simulink model "sampleModel1420_5"  (R2023a)
settings: Solver=VariableStepAuto  StartTime=0.0  StopTime=10.0  RelTol=1e-3
libraries: hdlsllib x5, simulink x2
settings Model: Creator=user1  LastModifiedBy=user1

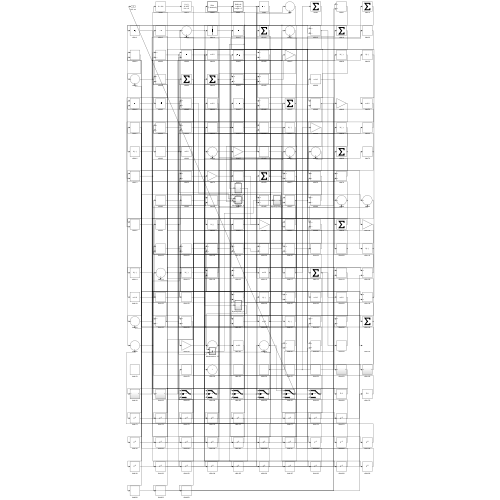
[thumbnail: Simulink's stored preview of the top-level diagram]
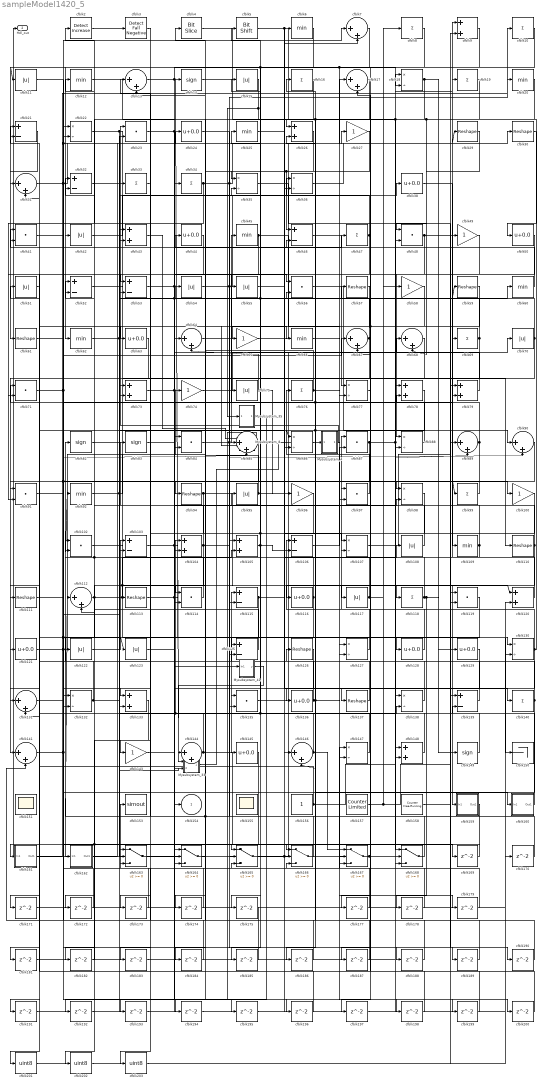
== system sampleModel1420_5 ==
  Mysubsystem_33 : Subsystem  TreatAsAtomicUnit=on  RTWFcnName=Mysubsystem_33
      settings: RTWFcnNameOpts=User specified  RTWFileNameOpts=Use function name
  Mysubsystem_35 : Subsystem  TreatAsAtomicUnit=on  RTWFcnName=Mysubsystem_35
      settings: RTWFcnNameOpts=User specified  RTWFileNameOpts=Use function name
  Mysubsystem_4 : Subsystem  TreatAsAtomicUnit=on  RTWFcnName=Mysubsystem_4
      settings: RTWFcnNameOpts=User specified  RTWFileNameOpts=Use function name
  Mysubsystem_41 : Subsystem  TreatAsAtomicUnit=on  RTWFcnName=Mysubsystem_41
      settings: RTWFcnNameOpts=User specified  RTWFileNameOpts=Use function name
  Mysubsystem_8 : Subsystem  TreatAsAtomicUnit=on  RTWFcnName=Mysubsystem_8
      settings: RTWFcnNameOpts=User specified  RTWFileNameOpts=Use function name
  cfblk{8,10,16,19,33..34,47,69,76,99,118,140} (12 alike) : Sum  Inputs=+  OutDataTypeStr=uint8
  cfblk{27,49,58,65,74,96,100,143} (8 alike) : Gain  OutDataTypeStr=uint8
  cfblk{23,41,48,56,71,84,87,91,97,102,114,119,135} (13 alike) : DotProduct  OutDataTypeStr=uint8
  cfblk{21,32,46,52..53,103,106,115,125,139} (10 alike) : Sum  Inputs=+-  OutDataTypeStr=uint8
  cfblk{9,26,43,73,78..79,104..105,120,133,148} (11 alike) : Sum  OutDataTypeStr=uint8
  cfblk{18,22,35..36,77,86,88,98,107,127,130,132,138,147} (14 alike) : Product  Inputs=*/  OutDataTypeStr=uint8  RndMeth=Zero  SaturateOnIntegerOverflow=on
  cfblk{11,15,42,51,54..55,70,75,95,108,117,122..123} (13 alike) : Abs  OutDataTypeStr=uint8  SaturateOnIntegerOverflow=off
  cfblk{6,12,20,25,45,60,62,66,92,109} (10 alike) : MinMax  OutDataTypeStr=uint8
  cfblk{29..30,57,59,61,94,110..111,113,126,137} (11 alike) : Reshape
  cfblk{7,13,17,31,64,67..68,85,89..90,112,131,141,144,146} (15 alike) : Sum  Inputs=|++  OutDataTypeStr=uint8
  cfblk{24,38,44,50,63,116,121,128..129,136,145} (11 alike) : Bias  Bias=0.0  SaturateOnIntegerOverflow=off
  cfblk{14,82..83,149} (4 alike) : Signum
  cfblk150 : Terminator
  cfblk151 : Scope
      settings: Floating=on
  cfblk153 : ToWorkspace  VariableName=simout  SaveFormat=Timeseries  SampleTime=-1
  cfblk155 : Scope
      settings: Floating=on
  cfblk156 : Constant  OutDataTypeStr=uint8  SampleTime=-1
  cfblk157 : hdlsllib/Sources/Counter Limited  uplimit=7  tsamp=-1
  cfblk158 : hdlsllib/Sources/Counter Free-Running  NumBits=16  tsamp=-1
  cfblk159 : Subsystem
      settings: LibrarySourceBlock=|
      | hdlsllib/Ports &
      | Subsystems/Subsystem
  cfblk160 : Subsystem
      settings: LibrarySourceBlock=|
      | hdlsllib/Ports &
      | Subsystems/Subsystem
  cfblk161 : Subsystem
      settings: LibrarySourceBlock=|
      | hdlsllib/Ports &
      | Subsystems/Subsystem
  cfblk162 : Subsystem
      settings: LibrarySourceBlock=|
      | hdlsllib/Ports &
      | Subsystems/Subsystem
  cfblk{163..168} (6 alike) : Switch  OutDataTypeStr=uint8  SaturateOnIntegerOverflow=off  InputSameDT=off
  cfblk{169..175,177..179,181..200} (30 alike) : Delay  SampleTime=1
  cfblk2 : simulink/Logic and Bit Operations/Detect Increase  vinit=0.0  OutDataTypeStr=uint8
      settings: LibrarySourceBlock=|
      | hdlsllib/Logic and Bit
      | Operations/Detect
      | Increase
  cfblk201 : DataTypeConversion  OutDataTypeStr=uint8  SaturateOnIntegerOverflow=off  RndMeth=Floor
  cfblk202 : DataTypeConversion  OutDataTypeStr=uint8  SaturateOnIntegerOverflow=off  RndMeth=Floor
  cfblk203 : DataTypeConversion  OutDataTypeStr=uint8  SaturateOnIntegerOverflow=off  RndMeth=Floor
  cfblk3 : hdlsllib/Logic and Bit Operations/Detect Fall Negative  vinit=0  OutDataTypeStr=uint8
  cfblk4 : hdlsllib/Logic and Bit Operations/Bit Slice  lidx=7  ridx=0
  cfblk5 : hdlsllib/Logic and Bit Operations/Bit Shift  mode=Shift Left Logical  N=0
  cfblk154 : Outport  OutDataTypeStr=uint8  VectorParamsAs1DForOutWhenUnconnected=off
  Hdl_out : Outport  Port=2  OutDataTypeStr=uint8
  wires:
  cfblk165/1 -> cfblk70/1, cfblk108/1
  cfblk140/1 -> cfblk153/1, cfblk126/1
  cfblk144/1 -> cfblk166/1, cfblk41/2
  cfblk139/1 -> cfblk115/1
  cfblk6/1 -> cfblk61/1
  cfblk75/1 -> cfblk96/1, cfblk64/2
  cfblk162/1(Out1) -> cfblk27/1
  cfblk59/1 -> Mysubsystem_8/2(In2), cfblk197/1
  cfblk54/1 -> cfblk38/1, cfblk188/1
  cfblk138/1 -> cfblk82/1
  cfblk161/1(Out1) -> cfblk10/1
  cfblk62/1 -> cfblk130/1, cfblk60/1
  cfblk94/1 -> cfblk159/1(In1), cfblk183/1
  cfblk10/1 -> cfblk62/1
  cfblk127/1 -> cfblk87/1
  cfblk130/1 -> cfblk26/1, cfblk164/3, cfblk67/2
  cfblk115/1 -> cfblk162/1(In1), cfblk7/2
  cfblk22/1 -> cfblk118/1, cfblk86/2
  cfblk70/1 -> cfblk141/1, cfblk53/2
  cfblk48/1 -> cfblk88/1, cfblk190/1
  cfblk23/1 -> cfblk144/1, cfblk167/3
  cfblk116/1 -> cfblk43/1, cfblk191/1
  cfblk63/1 -> cfblk161/1(In1)
  cfblk97/1 -> cfblk76/1
  cfblk146/1 -> cfblk25/1, cfblk21/1, cfblk167/1
  cfblk56/1 -> cfblk90/1
  cfblk148/1 -> cfblk104/1, cfblk43/2
  cfblk121/1 -> cfblk74/1, cfblk67/1
  cfblk16/1 -> cfblk53/1
  cfblk110/1 -> cfblk83/1, cfblk136/1
  cfblk95/1 -> cfblk44/1, cfblk98/1
  cfblk4/1 -> cfblk127/1
  cfblk168/1 -> cfblk112/1, cfblk114/2
  cfblk87/1 -> cfblk89/2, cfblk19/1, cfblk175/1
  cfblk5/1 -> cfblk168/1, cfblk107/1
  cfblk117/1 -> cfblk92/1, cfblk2/1, cfblk58/1
  cfblk26/1 -> cfblk165/1
  cfblk109/1 -> cfblk97/1, cfblk107/2
  cfblk85/1 -> cfblk121/1
  cfblk46/1 -> cfblk77/1
  cfblk120/1 -> cfblk9/1
  cfblk104/1 -> cfblk73/2, cfblk122/1, cfblk20/1
  cfblk50/1 -> cfblk85/1
  cfblk88/1 -> cfblk45/1
  cfblk57/1 -> cfblk91/1
  cfblk12/1 -> cfblk64/1
  cfblk51/1 -> cfblk131/1
  cfblk125/1 -> cfblk71/1
  cfblk106/1 -> cfblk87/2
  cfblk65/1 -> cfblk17/1
  cfblk2/1 -> cfblk3/1
  cfblk67/1 -> cfblk115/2, cfblk15/1
  cfblk112/1 -> cfblk147/2, cfblk34/1, cfblk12/1
  cfblk122/1 -> cfblk103/1
  cfblk34/1 -> cfblk55/1, cfblk18/1, cfblk71/2
  cfblk11/1 -> cfblk164/2
  cfblk38/1 -> cfblk109/1
  cfblk149/1 -> cfblk54/1
  cfblk64/1 -> cfblk66/1
  cfblk17/1 -> cfblk146/2, cfblk173/1
  cfblk47/1 -> cfblk91/2, cfblk13/1
  cfblk123/1 -> cfblk154/1
  cfblk163/1 -> cfblk105/2
  cfblk156/1 -> cfblk131/2, cfblk48/2
  cfblk90/1 -> cfblk132/2
  cfblk31/1 -> cfblk14/1, cfblk7/1
  cfblk158/1 -> cfblk139/1
  cfblk45/1 -> cfblk97/2, cfblk103/2
  cfblk159/1(Out1) -> cfblk181/1, cfblk182/1
  cfblk27/1 -> cfblk46/1, cfblk184/1
  cfblk108/1 -> cfblk52/1
  cfblk83/1 -> cfblk36/1, cfblk59/1
  cfblk103/1 -> cfblk150/1, cfblk57/1
  cfblk86/1 -> cfblk100/1
  cfblk113/1 -> cfblk128/1, cfblk98/2
  cfblk84/1 -> cfblk90/2, cfblk79/2
  cfblk166/1 -> cfblk33/1
  cfblk15/1 -> Mysubsystem_35/1(In1), cfblk193/1
  cfblk135/1 -> cfblk137/1
  cfblk36/1 -> cfblk30/1
  cfblk92/1 -> cfblk24/1, cfblk167/2
  cfblk132/1 -> cfblk51/1, cfblk138/2
  cfblk29/1 -> cfblk48/1
  cfblk76/1 -> cfblk13/2, cfblk179/1
  cfblk79/1 -> cfblk65/1
  cfblk105/1 -> cfblk5/1, cfblk106/2
  cfblk61/1 -> cfblk123/1, cfblk160/1(In1), cfblk99/1
  cfblk102/1 -> cfblk145/1, cfblk120/1
  cfblk98/1 -> cfblk135/1, cfblk125/2
  cfblk69/1 -> cfblk4/1, cfblk35/2, cfblk194/1
  cfblk21/1 -> cfblk31/1
  cfblk73/1 -> cfblk69/1, cfblk195/1
  cfblk58/1 -> cfblk78/1
  cfblk167/1 -> cfblk138/1, Hdl_out/1
  cfblk141/1 -> cfblk163/2, cfblk113/1
  cfblk74/1 -> cfblk68/1
  cfblk52/1 -> cfblk110/1
  cfblk71/1 -> cfblk22/2, cfblk29/1, cfblk85/2
  cfblk82/1 -> cfblk75/1
  cfblk164/1 -> cfblk84/2
  cfblk33/1 -> cfblk63/1
  cfblk107/1 -> cfblk49/1
  cfblk30/1 -> cfblk50/1
  cfblk53/1 -> cfblk56/1, cfblk199/1
  cfblk131/1 -> cfblk78/2
  cfblk99/1 -> cfblk94/1
  cfblk96/1 -> cfblk133/1
  cfblk128/1 -> cfblk106/1
  cfblk13/1 -> Mysubsystem_41/1(In1), cfblk18/2
  cfblk114/1 -> cfblk52/2
  cfblk25/1 -> cfblk140/1
  cfblk19/1 -> cfblk125/1, cfblk68/2
  cfblk143/1 -> cfblk47/1
  cfblk89/1 -> cfblk32/1, cfblk56/2, cfblk135/2
  cfblk20/1 -> cfblk88/2, cfblk114/1
  cfblk9/1 -> cfblk11/1, cfblk35/1, cfblk127/2
  cfblk147/1 -> cfblk102/1
  cfblk24/1 -> cfblk77/2
  cfblk18/1 -> cfblk42/1, cfblk129/1
  cfblk68/1 -> cfblk86/1, cfblk116/1
  cfblk44/1 -> cfblk111/1
  cfblk35/1 -> cfblk89/1
  cfblk42/1 -> cfblk6/1
  cfblk100/1 -> cfblk143/1
  cfblk41/1 -> cfblk133/2
  cfblk136/1 -> cfblk16/1, cfblk200/1, cfblk95/1
  cfblk160/1(Out1) -> cfblk139/2
  cfblk60/1 -> cfblk41/1
  cfblk14/1 -> cfblk148/1
  cfblk55/1 -> cfblk36/2
  cfblk118/1 -> cfblk149/1, cfblk178/1, cfblk32/2
  cfblk157/1 -> cfblk9/2, cfblk8/1
  cfblk8/1 -> cfblk117/1
  cfblk137/1 -> cfblk46/2
  cfblk66/1 -> cfblk169/1
  cfblk169/1 -> cfblk165/2
  cfblk170/1 -> cfblk105/1
  cfblk78/1 -> cfblk171/1
  cfblk171/1 -> cfblk130/2
  cfblk133/1 -> cfblk172/1
  cfblk172/1 -> cfblk132/1
  cfblk173/1 -> cfblk163/1
  cfblk126/1 -> cfblk174/1
  cfblk174/1 -> cfblk112/2
  cfblk175/1 -> cfblk141/2
  cfblk77/1 -> cfblk177/1
  cfblk177/1 -> cfblk166/3
  cfblk178/1 -> cfblk147/1
  cfblk179/1 -> cfblk165/3
  cfblk181/1 -> cfblk144/2
  cfblk182/1 -> cfblk102/2
  cfblk183/1 -> cfblk148/2
  cfblk184/1 -> cfblk163/3
  cfblk7/1 -> cfblk185/1
  cfblk185/1 -> cfblk22/1
  cfblk129/1 -> cfblk186/1
  cfblk186/1 -> cfblk84/1
  cfblk49/1 -> cfblk187/1
  cfblk187/1 -> cfblk26/2
  cfblk188/1 -> cfblk104/2
  cfblk91/1 -> cfblk189/1
  cfblk189/1 -> cfblk73/1
  cfblk190/1 -> cfblk21/2
  cfblk191/1 -> cfblk164/1
  cfblk192/1 -> cfblk23/2
  cfblk193/1 -> cfblk120/2
  cfblk194/1 -> cfblk79/1
  cfblk195/1 -> cfblk146/1
  cfblk196/1 -> cfblk166/2
  cfblk197/1 -> cfblk168/3
  cfblk111/1 -> cfblk198/1
  cfblk198/1 -> cfblk168/2
  cfblk199/1 -> cfblk17/2
  cfblk200/1 -> cfblk31/2
  cfblk119/1 -> cfblk201/1
  cfblk201/1 -> cfblk170/1
  cfblk145/1 -> cfblk202/1
  cfblk202/1 -> cfblk119/1
  cfblk3/1 -> cfblk203/1
  cfblk203/1 -> cfblk119/2
  Mysubsystem_4/1(Out1) -> cfblk23/1
  cfblk43/1 -> Mysubsystem_8/1(In1)
  Mysubsystem_8/1(Out1) -> cfblk196/1
  cfblk32/1 -> Mysubsystem_33/2(In2)
  Mysubsystem_33/1(Out1) -> Mysubsystem_4/1(In1)
  Mysubsystem_35/1(Out1) -> cfblk192/1
  Mysubsystem_41/1(y) -> Mysubsystem_33/1(In1)

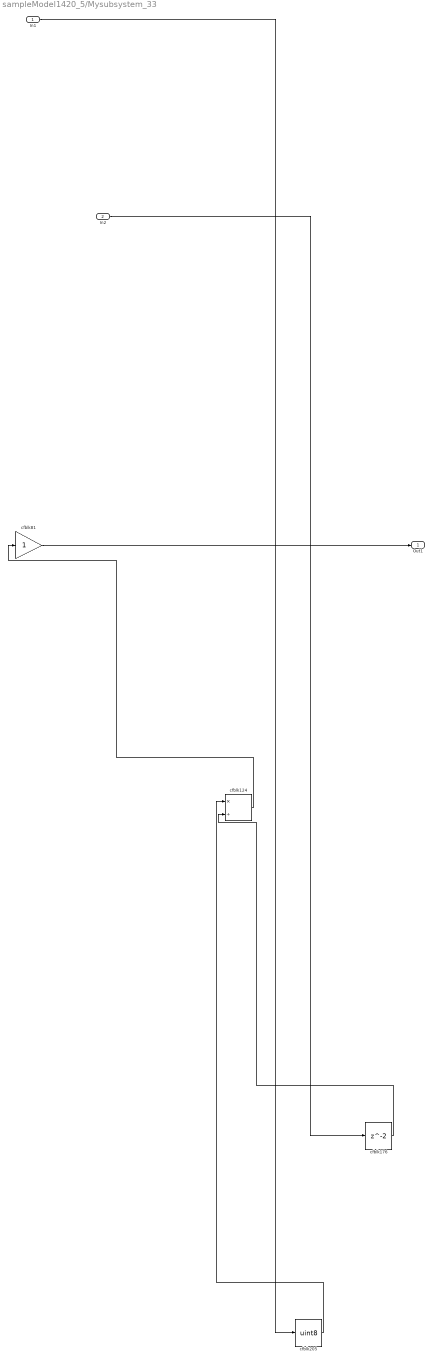
== system sampleModel1420_5/Mysubsystem_33 ==
  In1 : Inport
  In2 : Inport  Port=2
  cfblk124 : Product  Inputs=*/  RndMeth=Zero  SaturateOnIntegerOverflow=on
  cfblk176 : Delay  SampleTime=1
  cfblk205 : DataTypeConversion  OutDataTypeStr=uint8  SaturateOnIntegerOverflow=off  RndMeth=Floor
  cfblk81 : Gain
  Out1 : Outport
  wires:
  cfblk81/1 -> Out1/1
  cfblk205/1 -> cfblk124/1
  In2/1 -> cfblk176/1
  cfblk176/1 -> cfblk124/2
  cfblk124/1 -> cfblk81/1
  In1/1 -> cfblk205/1

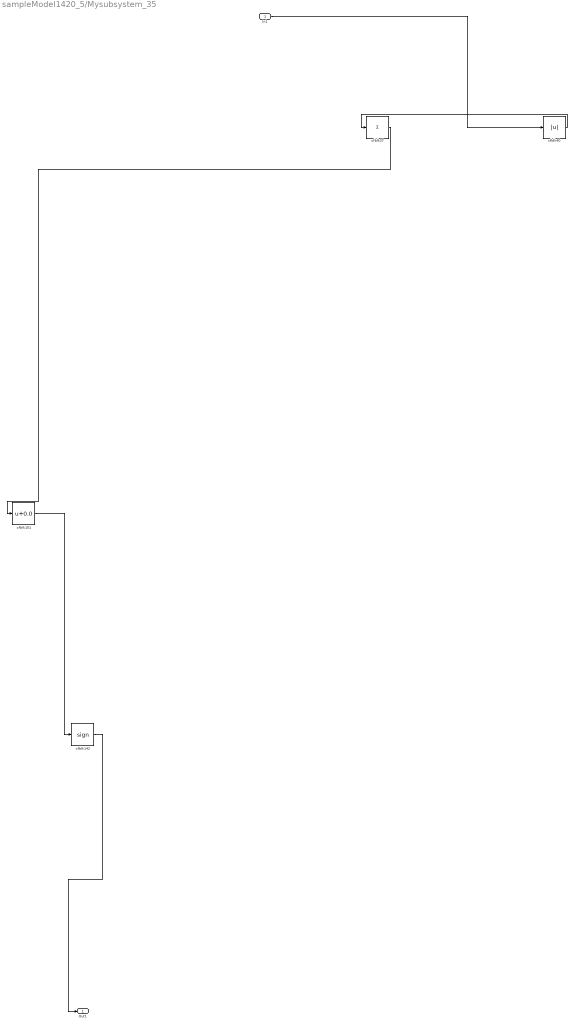
== system sampleModel1420_5/Mysubsystem_35 ==
  In1 : Inport
  cfblk101 : Bias  Bias=0.0  SaturateOnIntegerOverflow=off
  cfblk142 : Signum
  cfblk37 : Sum  Inputs=+
  cfblk40 : Abs  SaturateOnIntegerOverflow=off
  Out1 : Outport
  wires:
  cfblk37/1 -> cfblk101/1
  In1/1 -> cfblk40/1
  cfblk40/1 -> cfblk37/1
  cfblk101/1 -> cfblk142/1
  cfblk142/1 -> Out1/1

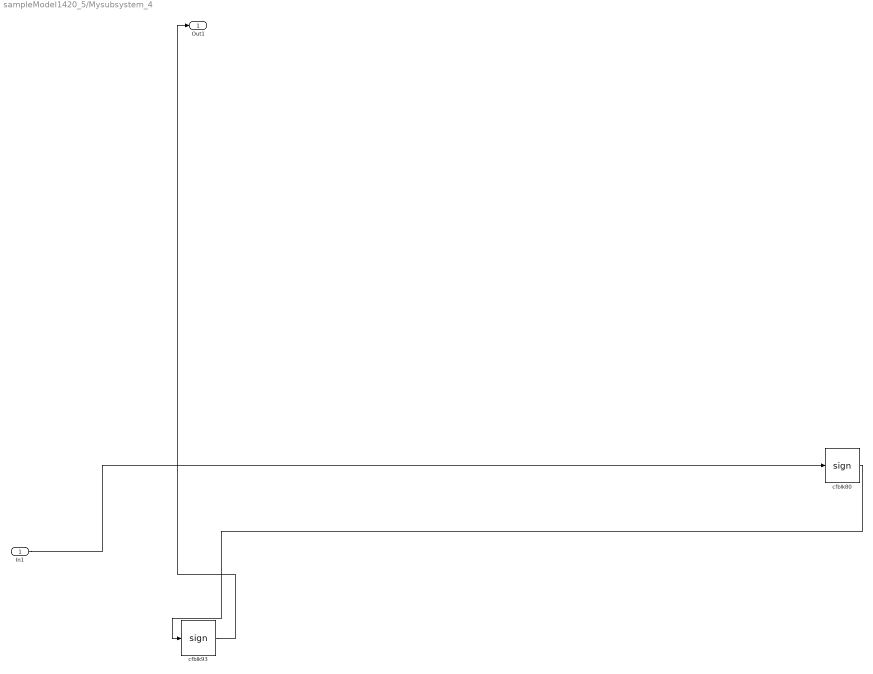
== system sampleModel1420_5/Mysubsystem_4 ==
  In1 : Inport
  cfblk80 : Signum
  cfblk93 : Signum
  Out1 : Outport
  wires:
  In1/1 -> cfblk80/1
  cfblk80/1 -> cfblk93/1
  cfblk93/1 -> Out1/1

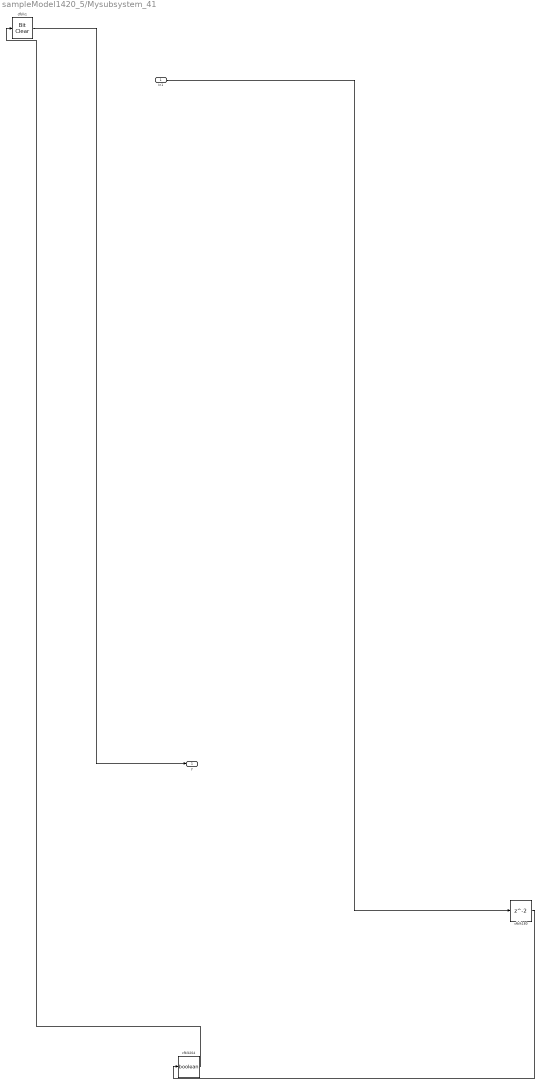
== system sampleModel1420_5/Mysubsystem_41 ==
  In1 : Inport
  cfblk1 : simulink/Logic and Bit Operations/Bit Clear  iBit=0
      settings: LibrarySourceBlock=|
      | hdlsllib/Logic and Bit
      | Operations/Bit Clear
  cfblk180 : Delay  SampleTime=1
  cfblk204 : DataTypeConversion  OutDataTypeStr=boolean  SaturateOnIntegerOverflow=off  RndMeth=Floor
  y : Outport
  wires:
  In1/1 -> cfblk180/1
  cfblk204/1 -> cfblk1/1
  cfblk180/1 -> cfblk204/1
  cfblk1/1 -> y/1

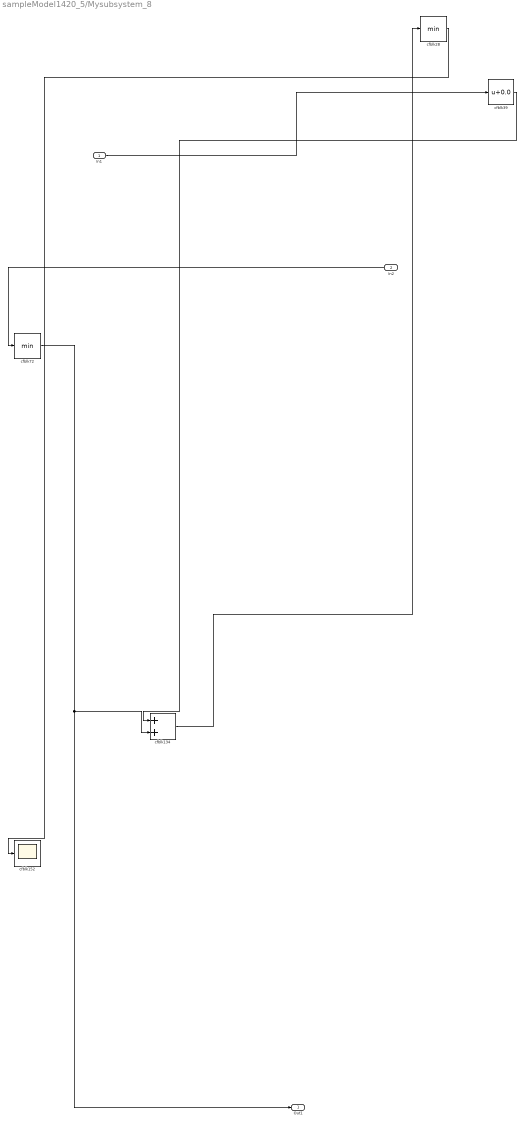
== system sampleModel1420_5/Mysubsystem_8 ==
  In1 : Inport
  In2 : Inport  Port=2
  cfblk134 : Sum
  cfblk152 : Scope
  cfblk28 : MinMax
  cfblk39 : Bias  Bias=0.0  SaturateOnIntegerOverflow=off
  cfblk72 : MinMax
  Out1 : Outport
  wires:
  cfblk28/1 -> cfblk152/1
  In1/1 -> cfblk39/1
  In2/1 -> cfblk72/1
  cfblk72/1 -> Out1/1, cfblk134/2
  cfblk134/1 -> cfblk28/1
  cfblk39/1 -> cfblk134/1

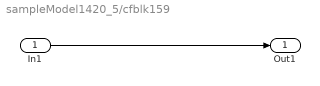
== system sampleModel1420_5/cfblk159 ==
  In1 : Inport
  Out1 : Outport
  wires:
  In1/1 -> Out1/1

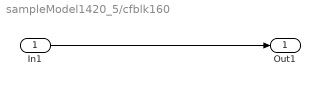
== system sampleModel1420_5/cfblk160 ==
  In1 : Inport
  Out1 : Outport
  wires:
  In1/1 -> Out1/1

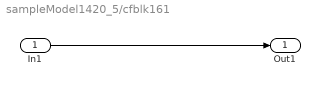
== system sampleModel1420_5/cfblk161 ==
  In1 : Inport
  Out1 : Outport
  wires:
  In1/1 -> Out1/1

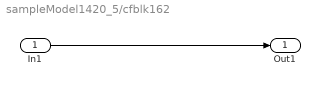
== system sampleModel1420_5/cfblk162 ==
  In1 : Inport
  Out1 : Outport
  wires:
  In1/1 -> Out1/1
